simulink model "ClosedLoop"  (R2018b)
settings: Solver=VariableStepAuto  StartTime=0.0  StopTime=10.0  RelTol=1e-3
settings Model: Creator=manzand  LastModifiedBy=manzand

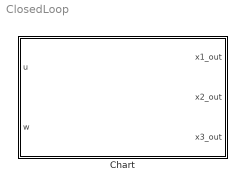
== system ClosedLoop ==
  Chart : Stateflow chart  TreatAsAtomicUnit=on

== stateflow chart ClosedLoop/Chart ==
  settings: updateMethod=CONTINUOUS
  state b1
    du:
    x1_dot = x2 + 0.5*x3^2;
    x2_dot = x3 + w;
    x3_dot = u;
    % Outputs
    x1_out = x1;
    x2_out = x2;
    x3_out = x3;
  (default) -> b1
  data: u input; w input; x1_out output; x2_out output; x1 local; x2 local; x3 local; x3_out output
  data x1 settings: updateMethod=SF_CONTINUOUS_TIME_DATA
  data x2 settings: updateMethod=SF_CONTINUOUS_TIME_DATA
  data x3 settings: updateMethod=SF_CONTINUOUS_TIME_DATA
